simulink model "HumanoidModel_ResidualRL"  (R2025b)
settings: Solver=daessc  StartTime=0.0  StopTime=11  RelTol=1e-3  AbsTol=1e-3
PreLoadFcn:
  | addpath(fullfile('ImportedURDFSupport','Geometries'));
  | addpath(fullfile('ImportedURDFSupport','Data'));
undefined symbols (not defined in the file): kd_ankle_vy, kd_ankle_wx, kd_hip_sag_vx, kd_hip_sag_wy, kd_hip_vy, kd_hip_vz, kd_hip_wx, kp_ankle_qx, kp_ankle_y, kp_hip_dz, kp_hip_qx, kp_hip_sag_qy, kp_hip_sag_x, kp_hip_y, params, residualRLActionPenaltyWeight, residualRLActionRatePenaltyWeight, residualRLAliveReward, residualRLChannelMap, residualRLEnabled, residualRLLeftFootLoadMap, residualRLManualAction, residualRLNominalFootLoad_N, residualRLObservationInverseScales, residualRLRewardStateWeights, residualRLRightFootLoadMap, residualRLSampleTime_s, residualRLTerminalPenalty, residualRLTorqueLimit_Nm, residualRLUseAgent, robustnessForceDuration_s, robustnessForceStart_s, robustnessForceVector_N, Rx_ref, u_ankle_pitch, u_hip_frontal, u_hip_sagittal, u_knee, u_shoulder_frontal, X, Y, y_ref, Z
libraries: sm_lib x155, nesl_utility x96, simulink_extras x18, simulink x5, robotmaniplib x1, rllib x1
(part 6 of 6)

== system HumanoidModel_ResidualRL/Humanoid Robot/Legs/Right leg/Knee Joint ==
  note: lower leg
  note: upper leg
  Torque : Inport
  Bus Creator2 : BusCreator  Inputs=2
  Constant : Constant  Value=0
  Knee Axis Transform : sm_lib/Frames and Transforms/Rigid Transform  RotationMethod=ArbitraryAxis  FollAlignAxisA=+X  BaseAlignAxisA=+Y  FollAlignAxisB=+Y  BaseAlignAxisB=+Z  RotationStandardAxis=+Z  RotationAngle=1.570796326794897  RotationAngleUnits=rad  RotationArbitraryAxis=[-0, 1, 0]  RotationSequenceAxes=FollowerAxes  RotationSequence=XYX  RotationSequenceAngles=[0 0 0]  RotationSequenceAnglesUnits=deg  RotationMatrix=[1 0 0; 0 1 0; 0 0 1]  Quaternion=[1 0 0 0]  TranslationMethod=Cartesian  TranslationCartesianOffset=[0, 0, 0]  TranslationCartesianOffsetUnits=m  TranslationStandardAxis=+Z  TranslationStandardOffset=0  TranslationStandardOffsetUnits=m  TranslationROffset=0  TranslationROffsetUnits=m  TranslationThetaOffset=0  TranslationThetaOffsetUnits=deg  TranslationZOffset=0  TranslationZOffsetUnits=m
  Knee Axis Transform Reverse : sm_lib/Frames and Transforms/Rigid Transform  RotationMethod=ArbitraryAxis  FollAlignAxisA=+X  BaseAlignAxisA=+Y  FollAlignAxisB=+Y  BaseAlignAxisB=+Z  RotationStandardAxis=+Z  RotationAngle=1.570796326794897  RotationAngleUnits=rad  RotationArbitraryAxis=[-0, -1, 0]  RotationSequenceAxes=FollowerAxes  RotationSequence=XYX  RotationSequenceAngles=[0 0 0]  RotationSequenceAnglesUnits=deg  RotationMatrix=[1 0 0; 0 1 0; 0 0 1]  Quaternion=[1 0 0 0]  TranslationMethod=Cartesian  TranslationCartesianOffset=[0, 0, 0]  TranslationCartesianOffsetUnits=m  TranslationStandardAxis=+Z  TranslationStandardOffset=0  TranslationStandardOffsetUnits=m  TranslationROffset=0  TranslationROffsetUnits=m  TranslationThetaOffset=0  TranslationThetaOffsetUnits=deg  TranslationZOffset=0  TranslationZOffsetUnits=m
  Knee Origin Transform : sm_lib/Frames and Transforms/Rigid Transform  RotationMethod=RotationSequence  FollAlignAxisA=+X  BaseAlignAxisA=+Y  FollAlignAxisB=+Y  BaseAlignAxisB=+Z  RotationStandardAxis=+Z  RotationAngle=0.0  RotationAngleUnits=deg  RotationArbitraryAxis=[0 0 1]  RotationSequenceAxes=BaseAxes  RotationSequence=XYZ  RotationSequenceAngles=[0, 0, 0]  RotationSequenceAnglesUnits=rad  RotationMatrix=[1 0 0; 0 1 0; 0 0 1]  Quaternion=[1 0 0 0]  TranslationMethod=Cartesian  TranslationCartesianOffset=[-0.02537, 0, -0.1041]*3.5  TranslationCartesianOffsetUnits=m  TranslationStandardAxis=+Z  TranslationStandardOffset=0  TranslationStandardOffsetUnits=m  TranslationROffset=0  TranslationROffsetUnits=m  TranslationThetaOffset=0  TranslationThetaOffsetUnits=deg  TranslationZOffset=0  TranslationZOffsetUnits=m
  PS-Simulink Converter2 : nesl_utility/PS-Simulink Converter  PhysicalDomain=network_engine_domain  SubClassName=ps_output  LeftPortType=input  RightPortType=output  PseudoPeriodic=off  Frequencies=[]  VectorFormat=1-D array  Unit=inherit  AffineConversion=off
  PS-Simulink Converter3 : nesl_utility/PS-Simulink Converter  PhysicalDomain=network_engine_domain  SubClassName=ps_output  LeftPortType=input  RightPortType=output  PseudoPeriodic=off  Frequencies=[]  VectorFormat=1-D array  Unit=inherit  AffineConversion=off
  Simulink-PS Converter1 : nesl_utility/Simulink-PS Converter  PhysicalDomain=network_engine_domain  SubClassName=ps_input  LeftPortType=input  RightPortType=output  PseudoPeriodic=off  Frequencies=[]  NoiseDistribution=none  NoiseParameters=[]  Unit=N*m  AffineConversion=off  FilteringAndDerivatives=provide  SimscapeFilterOrder=1  InputFilterTimeConstant=0.001  UdotUserProvided=0
  Simulink-PS Converter3 : nesl_utility/Simulink-PS Converter  PhysicalDomain=network_engine_domain  SubClassName=ps_input  LeftPortType=input  RightPortType=output  PseudoPeriodic=off  Frequencies=[]  NoiseDistribution=none  NoiseParameters=[]  Unit=rad  AffineConversion=off  FilteringAndDerivatives=provide  SimscapeFilterOrder=1  InputFilterTimeConstant=0.001  UdotUserProvided=0
  right_knee : sm_lib/Joints/Revolute Joint  JointMode=Normal  CompositeWrenchDir=FollowerOnBase  CompositeWrenchFrame=BaseFrame  SenseConstraintForce=off  SenseConstraintTorque=off  SenseTotalForce=off  SenseTotalTorque=off  PositionTargetSpecify=on  PositionTargetPriority=High  PositionTargetValue=30  PositionTargetValueUnits=deg  VelocityTargetSpecify=off  VelocityTargetPriority=High  VelocityTargetValue=0  VelocityTargetValueUnits=deg/s  EquilibriumPosition=0  EquilibriumPositionUnits=deg  SpringStiffness=0  SpringStiffnessUnits=N*m/deg  DampingCoefficient=2.5  DampingCoefficientUnits=m^2*kg/s/rad  LowerLimitSpecify=on  LowerLimitBound=kneeLowerLimit  LowerLimitBoundUnits=deg  LowerLimitStiffness=1e4  LowerLimitStiffnessUnits=N*m/deg  LowerLimitDamping=10  LowerLimitDampingUnits=N*m/(deg/s)  LowerLimitTransitionRegionWidth=0.1  LowerLimitTransitionRegionWidthUnits=deg  UpperLimitSpecify=on  UpperLimitBound=kneeUpperLimit  UpperLimitBoundUnits=deg  UpperLimitStiffness=1e4  UpperLimitStiffnessUnits=N*m/deg  UpperLimitDamping=10  UpperLimitDampingUnits=N*m/(deg/s)  UpperLimitTransitionRegionWidth=0.1  UpperLimitTransitionRegionWidthUnits=deg  TorqueActuationMode=InputTorque  MotionActuationMode=ComputedMotion  SensePosition=on  SenseVelocity=on  SenseAcceleration=off  SenseTorqueForce=off  SenseLowerLimitTorqueForce=off  SenseUpperLimitTorqueForce=off
  "F1 " : PMIOPort  Side=Right
  F : PMIOPort  Port=2  Side=Left
  Sensing : Outport
  wires:
  Torque/1 -> Simulink-PS Converter1/1
  Bus Creator2/1 -> Sensing/1
  PS-Simulink Converter2/1 -> Bus Creator2/1  "rkTheta"
  PS-Simulink Converter3/1 -> Bus Creator2/2  "rkThetaDot"
  Constant/1 -> Simulink-PS Converter3/1
  connections:
  F/RConn1 -- Knee Origin Transform/LConn1
  Knee Axis Transform Reverse/RConn1 -- "F1 "/RConn1
  PS-Simulink Converter2/LConn1 -- right_knee/RConn2
  Knee Axis Transform/RConn1 -- right_knee/LConn1
  Knee Axis Transform/LConn1 -- Knee Origin Transform/RConn1
  PS-Simulink Converter3/LConn1 -- right_knee/RConn3
  Knee Axis Transform Reverse/LConn1 -- right_knee/RConn1
  Simulink-PS Converter1/RConn1 -- right_knee/LConn2
